simulink model "Roll_Autopilot_PP"  (R2017b)
settings: Solver=FixedStepDiscrete  StartTime=0.0  StopTime=10.0  FixedStep=0.025000  RelTol=1e-3
model workspace (MAT data in the model file):
  MCOS : class17 (value not decoded)
  already_pp = 1
  compositionalMap : struct (value not decoded)
  MCOS : class17 (value not decoded)
  MCOS : class17 (value not decoded)
  verificationResults : struct (value not decoded)
undefined symbols (not defined in the file): contractAfterSimulation, contractBeforeSimulation, ContractBlock, ContractEnsureBlock, ContractGuaranteeBlock, ContractModeBlock, ContractRequireBlock, ContractValidatorBlock, pp_lib, saturation, saveValidatorParameters, slcm, Ts
(part 3 of 3)

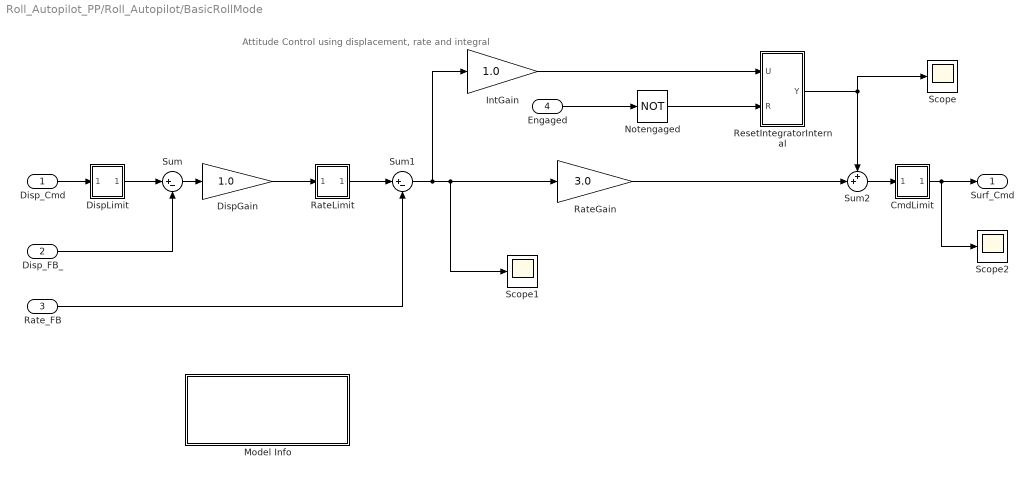
== system Roll_Autopilot_PP/Roll_Autopilot/BasicRollMode ==
  note: Attitude Control using displacement, rate and integral
  Disp_Cmd : Inport  OutDataTypeStr=double  PortDimensions=1
  Disp_FB_ : Inport  Port=2  OutDataTypeStr=double  PortDimensions=1  SampleTime=1/40
  Rate_FB : Inport  Port=3  OutDataTypeStr=double  PortDimensions=1  SampleTime=1/40
  Engaged : Inport  Port=4  OutDataTypeStr=boolean  PortDimensions=1  SampleTime=1/40
  CmdLimit : Subsystem  AncestorBlock=pp_lib/saturation  TreatAsAtomicUnit=on
  DispGain : Gain  Gain=1.0
  DispLimit : Subsystem  AncestorBlock=pp_lib/saturation  TreatAsAtomicUnit=on
  IntGain : Gain  Gain=1.0
  Model Info : Subsystem  AncestorBlock=simulink/Model-Wide Utilities/Model Info  LoadFcn=slcm LoadBlock;  InitFcn=slcm('UpdateAllCMBlocksInThisModelInit')  TreatAsAtomicUnit=on  mask(CMBlock){Frame=on, DisplayStringWithTags=|, MaskDisplayString=Attitude Controller\nAuthor: hbourbou\nVersion: 1.13\nDate: Wed Nov 06 15:53:17 2019, HorizontalTextAlignment=Left, LeftAlignmentValue=0.02}
      mask DisplayStringWithTags=|
      | Attitude Controller
      | Author: %<LastModifiedBy>
      | Version: %<ModelVersion>
      | Date: %<LastModificationDate>
      mask prompts: Frame "Simulink:masks:Frame_MP"; DisplayStringWithTags "Simulink:masks:DisplayStringWithTags_MP"; MaskDisplayString "Simulink:masks:MaskDisplayString_MP"; HorizontalTextAlignment "Simulink:masks:HorizontalTextAlignment_MP"; LeftAlignmentValue "Simulink:masks:LeftAlignmentValue_MP"
      mask help: Simulink:masks:CMBlock_MD
      settings: CopyFcn=slcm CopyBlock;  DeleteFcn=slcm Cancel;  PostSaveFcn=slcm('UpdateAllCMBlocksInThisModel')  NameChangeFcn=slcm Rename;  OpenFcn=slcm
      mask Display: text(slResolve(LeftAlignmentValue, gcbh), 0.5, MaskDisplayString, 'HorizontalAlignment', HorizontalTextAlignment)
  Notengaged : Logic  Operator=NOT  IconShape=distinctive  AllPortsSameDT=off  OutDataTypeStr=boolean
  RateGain : Gain  Gain=3.0
  RateLimit : Subsystem  AncestorBlock=pp_lib/saturation  TreatAsAtomicUnit=on
  ResetIntegratorInternal : Subsystem  TreatAsAtomicUnit=on
  Scope : Scope
  Scope1 : Scope
  Scope2 : Scope
  Sum : Sum  Inputs=|+-
  Sum1 : Sum  Inputs=|+-
  Sum2 : Sum  Inputs=++|
  Surf_Cmd : Outport  OutDataTypeStr=double  PortDimensions=1  SampleTime=1/40  VectorParamsAs1DForOutWhenUnconnected=off
  wires:
  Engaged/1 -> Notengaged/1
  Disp_Cmd/1 -> DispLimit/1(In)
  RateLimit/1(Out) -> Sum1/1
  ResetIntegratorInternal/1(Y) -> Sum2/1, Scope/1
  Notengaged/1 -> ResetIntegratorInternal/2(R)
  Rate_FB/1 -> Sum1/2
  Sum1/1 -> IntGain/1, Scope1/1, RateGain/1
  CmdLimit/1(Out) -> Scope2/1, Surf_Cmd/1
  RateGain/1 -> Sum2/2
  DispGain/1 -> RateLimit/1(In)
  Sum/1 -> DispGain/1
  Disp_FB_/1 -> Sum/2
  DispLimit/1(Out) -> Sum/1
  Sum2/1 -> CmdLimit/1(In)
  IntGain/1 -> ResetIntegratorInternal/1(U)

== system Roll_Autopilot_PP/Roll_Autopilot/HeadingMode ==
  PsiRef : Inport  OutDataTypeStr=double  PortDimensions=1  SampleTime=1/40  Interpolate=off
  Psi : Inport  Port=2  OutDataTypeStr=double  PortDimensions=1  SampleTime=1/40  Interpolate=off
  TAS : Inport  Port=3  OutDataTypeStr=double  PortDimensions=1  SampleTime=1/40  Interpolate=off
  DispGain : Gain  Gain=0.015
  Model Info : Subsystem  AncestorBlock=simulink/Model-Wide Utilities/Model Info  LoadFcn=slcm LoadBlock;  InitFcn=slcm('UpdateAllCMBlocksInThisModelInit')  TreatAsAtomicUnit=on  mask(CMBlock){Frame=on, DisplayStringWithTags=|, MaskDisplayString=Heading Mode\nAuthor: hbourbou\nVersion: 1.13\nDate: Wed Nov 06 15:53:17 2019, HorizontalTextAlignment=Left, LeftAlignmentValue=0.02}
      mask DisplayStringWithTags=|
      | Heading Mode
      | Author: %<LastModifiedBy>
      | Version: %<ModelVersion>
      | Date: %<LastModificationDate>
      mask prompts: Frame "Simulink:masks:Frame_MP"; DisplayStringWithTags "Simulink:masks:DisplayStringWithTags_MP"; MaskDisplayString "Simulink:masks:MaskDisplayString_MP"; HorizontalTextAlignment "Simulink:masks:HorizontalTextAlignment_MP"; LeftAlignmentValue "Simulink:masks:LeftAlignmentValue_MP"
      mask help: Simulink:masks:CMBlock_MD
      settings: CopyFcn=slcm CopyBlock;  DeleteFcn=slcm Cancel;  PostSaveFcn=slcm('UpdateAllCMBlocksInThisModel')  NameChangeFcn=slcm Rename;  OpenFcn=slcm
      mask Display: text(slResolve(LeftAlignmentValue, gcbh), 0.5, MaskDisplayString, 'HorizontalAlignment', HorizontalTextAlignment)
  Product : Product  RndMeth=Zero
  anglediff : Subsystem  TreatAsAtomicUnit=on
  PhiCmd : Outport  OutDataTypeStr=double  PortDimensions=1  SampleTime=1/40  VectorParamsAs1DForOutWhenUnconnected=off
  wires:
  PsiRef/1 -> anglediff/1(plus)
  anglediff/1(diff) -> DispGain/1  "hdgError"
  TAS/1 -> Product/2
  DispGain/1 -> Product/1
  Psi/1 -> anglediff/2(minus)
  Product/1 -> PhiCmd/1

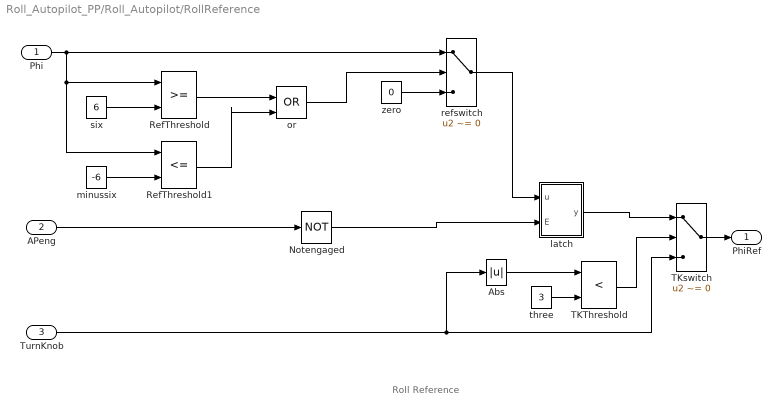
== system Roll_Autopilot_PP/Roll_Autopilot/RollReference ==
  note: Roll Reference
  Phi : Inport
  APeng : Inport  Port=2
  TurnKnob : Inport  Port=3
  Abs : Abs
  Notengaged : Logic  Operator=NOT  IconShape=distinctive  AllPortsSameDT=off  OutDataTypeStr=boolean
  RefThreshold : RelationalOperator  OutDataTypeStr=boolean  RndMeth=Nearest  InputSameDT=on
  RefThreshold1 : RelationalOperator  Operator=<=  OutDataTypeStr=boolean  RndMeth=Nearest  InputSameDT=on
  TKThreshold : RelationalOperator  Operator=<  OutDataTypeStr=boolean  RndMeth=Nearest  InputSameDT=on
  TKswitch : Switch  Criteria=u2 ~= 0
  latch : Subsystem  TreatAsAtomicUnit=on
  minussix : Constant  Value=-6
  or : Logic  Operator=OR  IconShape=distinctive  OutDataTypeStr=boolean
  refswitch : Switch  Criteria=u2 ~= 0
  six : Constant  Value=6
  three : Constant  Value=3  OutDataTypeStr=double
  zero : Constant  Value=0
  PhiRef : Outport  VectorParamsAs1DForOutWhenUnconnected=off
  wires:
  minussix/1 -> RefThreshold1/2
  RefThreshold1/1 -> or/2
  RefThreshold/1 -> or/1
  or/1 -> refswitch/2
  zero/1 -> refswitch/3
  six/1 -> RefThreshold/2
  TKswitch/1 -> PhiRef/1
  APeng/1 -> Notengaged/1
  Phi/1 -> RefThreshold1/1, RefThreshold/1, refswitch/1
  Abs/1 -> TKThreshold/1
  three/1 -> TKThreshold/2
  TurnKnob/1 -> Abs/1, TKswitch/3
  TKThreshold/1 -> TKswitch/2
  latch/1(y) -> TKswitch/1
  refswitch/1 -> latch/1(u)
  Notengaged/1 -> latch/2(E)

== system Roll_Autopilot_PP/Roll_Autopilot_RollAutopilotSpec1/AP_minus_001 ==
  In1 : Inport
  guarantee : Outport  OutDataTypeStr=boolean
  wires:
  In1/1 -> guarantee/1

== system Roll_Autopilot_PP/Roll_Autopilot_RollAutopilotSpec1/AP_minus_003A ==
  In1 : Inport
  guarantee : Outport  OutDataTypeStr=boolean
  wires:
  In1/1 -> guarantee/1

== system Roll_Autopilot_PP/Roll_Autopilot_RollAutopilotSpec1/AP_minus_003B ==
  In1 : Inport
  guarantee : Outport  OutDataTypeStr=boolean
  wires:
  In1/1 -> guarantee/1

== system Roll_Autopilot_PP/Roll_Autopilot_RollAutopilotSpec1/AP_minus_003C ==
  In1 : Inport
  guarantee : Outport  OutDataTypeStr=boolean
  wires:
  In1/1 -> guarantee/1

== system Roll_Autopilot_PP/Roll_Autopilot_RollAutopilotSpec1/AP_minus_003D ==
  In1 : Inport
  guarantee : Outport  OutDataTypeStr=boolean
  wires:
  In1/1 -> guarantee/1

== system Roll_Autopilot_PP/Roll_Autopilot_RollAutopilotSpec1/AP_minus_007 ==
  In1 : Inport
  guarantee : Outport  OutDataTypeStr=boolean
  wires:
  In1/1 -> guarantee/1

== system Roll_Autopilot_PP/Roll_Autopilot_RollAutopilotSpec1/H_call ==
  H_X : Inport  OutDataTypeStr=boolean
  Arrow_xxH_1_ni_23 : Delay  DelayLength=1  InitialCondition=1
  PRE_xxH_2 : Delay  DelayLength=1  InitialCondition=0
  branch_6_IF : Switch  Criteria=u2 ~= 0
  xxH_1_ni_23_init : Constant  Value=0  OutDataTypeStr=boolean
  xxH_3_operator : Logic  AllPortsSameDT=off  OutDataTypeStr=boolean
  H_Y : Outport
  wires:
  PRE_xxH_2/1 -> xxH_3_operator/2
  xxH_3_operator/1 -> branch_6_IF/3
  Arrow_xxH_1_ni_23/1 -> branch_6_IF/2
  xxH_1_ni_23_init/1 -> Arrow_xxH_1_ni_23/1
  branch_6_IF/1 -> H_Y/1, PRE_xxH_2/1
  H_X/1 -> xxH_3_operator/1, branch_6_IF/1

== system Roll_Autopilot_PP/Roll_Autopilot_RollAutopilotSpec1/H_call1 ==
  H_X : Inport  OutDataTypeStr=boolean
  Arrow_xxH_1_ni_23 : Delay  DelayLength=1  InitialCondition=1
  PRE_xxH_2 : Delay  DelayLength=1  InitialCondition=0
  branch_6_IF : Switch  Criteria=u2 ~= 0
  xxH_1_ni_23_init : Constant  Value=0  OutDataTypeStr=boolean
  xxH_3_operator : Logic  AllPortsSameDT=off  OutDataTypeStr=boolean
  H_Y : Outport
  wires:
  PRE_xxH_2/1 -> xxH_3_operator/2
  xxH_3_operator/1 -> branch_6_IF/3
  Arrow_xxH_1_ni_23/1 -> branch_6_IF/2
  xxH_1_ni_23_init/1 -> Arrow_xxH_1_ni_23/1
  branch_6_IF/1 -> H_Y/1, PRE_xxH_2/1
  H_X/1 -> xxH_3_operator/1, branch_6_IF/1

== system Roll_Autopilot_PP/Roll_Autopilot_RollAutopilotSpec1/H_call11 ==
  H_X : Inport  OutDataTypeStr=boolean
  Arrow_xxH_1_ni_23 : Delay  DelayLength=1  InitialCondition=1
  PRE_xxH_2 : Delay  DelayLength=1  InitialCondition=0
  branch_6_IF : Switch  Criteria=u2 ~= 0
  xxH_1_ni_23_init : Constant  Value=0  OutDataTypeStr=boolean
  xxH_3_operator : Logic  AllPortsSameDT=off  OutDataTypeStr=boolean
  H_Y : Outport
  wires:
  PRE_xxH_2/1 -> xxH_3_operator/2
  xxH_3_operator/1 -> branch_6_IF/3
  Arrow_xxH_1_ni_23/1 -> branch_6_IF/2
  xxH_1_ni_23_init/1 -> Arrow_xxH_1_ni_23/1
  branch_6_IF/1 -> H_Y/1, PRE_xxH_2/1
  H_X/1 -> xxH_3_operator/1, branch_6_IF/1

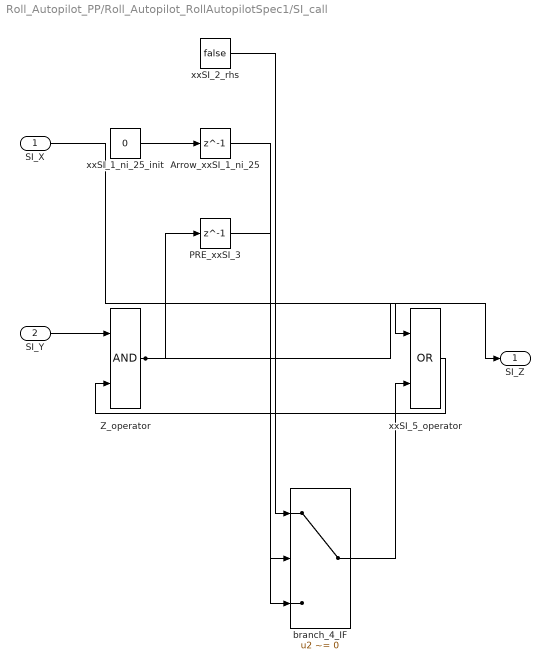
== system Roll_Autopilot_PP/Roll_Autopilot_RollAutopilotSpec1/SI_call ==
  SI_X : Inport  OutDataTypeStr=boolean
  SI_Y : Inport  Port=2  OutDataTypeStr=boolean
  Arrow_xxSI_1_ni_25 : Delay  DelayLength=1  InitialCondition=1
  PRE_xxSI_3 : Delay  DelayLength=1  InitialCondition=0
  Z_operator : Logic  AllPortsSameDT=off  OutDataTypeStr=boolean
  branch_4_IF : Switch  Criteria=u2 ~= 0
  xxSI_1_ni_25_init : Constant  Value=0  OutDataTypeStr=boolean
  xxSI_2_rhs : Constant  Value=false  OutDataTypeStr=boolean
  xxSI_5_operator : Logic  Operator=OR  AllPortsSameDT=off  OutDataTypeStr=boolean
  SI_Z : Outport
  wires:
  branch_4_IF/1 -> xxSI_5_operator/2
  SI_X/1 -> xxSI_5_operator/1
  PRE_xxSI_3/1 -> branch_4_IF/3
  Arrow_xxSI_1_ni_25/1 -> branch_4_IF/2
  xxSI_2_rhs/1 -> branch_4_IF/1
  xxSI_5_operator/1 -> Z_operator/2
  SI_Y/1 -> Z_operator/1
  xxSI_1_ni_25_init/1 -> Arrow_xxSI_1_ni_25/1
  Z_operator/1 -> SI_Z/1, PRE_xxSI_3/1

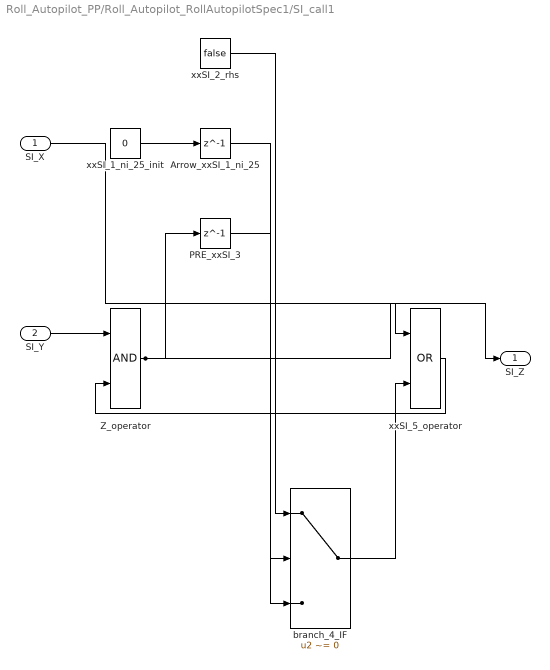
== system Roll_Autopilot_PP/Roll_Autopilot_RollAutopilotSpec1/SI_call1 ==
  SI_X : Inport  OutDataTypeStr=boolean
  SI_Y : Inport  Port=2  OutDataTypeStr=boolean
  Arrow_xxSI_1_ni_25 : Delay  DelayLength=1  InitialCondition=1
  PRE_xxSI_3 : Delay  DelayLength=1  InitialCondition=0
  Z_operator : Logic  AllPortsSameDT=off  OutDataTypeStr=boolean
  branch_4_IF : Switch  Criteria=u2 ~= 0
  xxSI_1_ni_25_init : Constant  Value=0  OutDataTypeStr=boolean
  xxSI_2_rhs : Constant  Value=false  OutDataTypeStr=boolean
  xxSI_5_operator : Logic  Operator=OR  AllPortsSameDT=off  OutDataTypeStr=boolean
  SI_Z : Outport
  wires:
  branch_4_IF/1 -> xxSI_5_operator/2
  SI_X/1 -> xxSI_5_operator/1
  PRE_xxSI_3/1 -> branch_4_IF/3
  Arrow_xxSI_1_ni_25/1 -> branch_4_IF/2
  xxSI_2_rhs/1 -> branch_4_IF/1
  xxSI_5_operator/1 -> Z_operator/2
  SI_Y/1 -> Z_operator/1
  xxSI_1_ni_25_init/1 -> Arrow_xxSI_1_ni_25/1
  Z_operator/1 -> SI_Z/1, PRE_xxSI_3/1

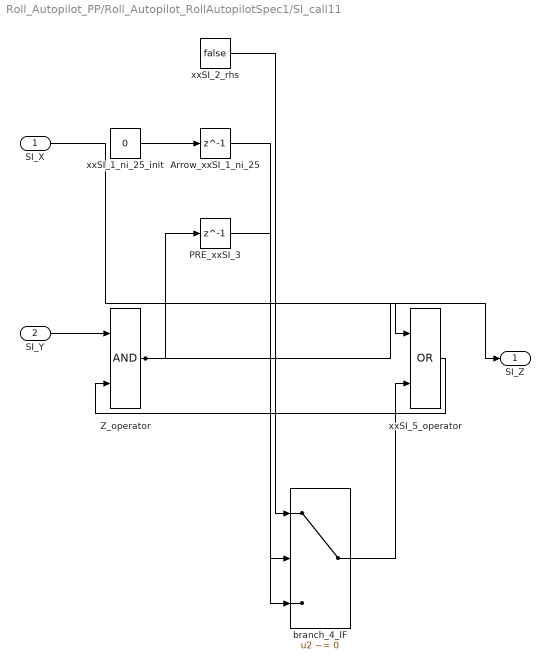
== system Roll_Autopilot_PP/Roll_Autopilot_RollAutopilotSpec1/SI_call11 ==
  SI_X : Inport  OutDataTypeStr=boolean
  SI_Y : Inport  Port=2  OutDataTypeStr=boolean
  Arrow_xxSI_1_ni_25 : Delay  DelayLength=1  InitialCondition=1
  PRE_xxSI_3 : Delay  DelayLength=1  InitialCondition=0
  Z_operator : Logic  AllPortsSameDT=off  OutDataTypeStr=boolean
  branch_4_IF : Switch  Criteria=u2 ~= 0
  xxSI_1_ni_25_init : Constant  Value=0  OutDataTypeStr=boolean
  xxSI_2_rhs : Constant  Value=false  OutDataTypeStr=boolean
  xxSI_5_operator : Logic  Operator=OR  AllPortsSameDT=off  OutDataTypeStr=boolean
  SI_Z : Outport
  wires:
  branch_4_IF/1 -> xxSI_5_operator/2
  SI_X/1 -> xxSI_5_operator/1
  PRE_xxSI_3/1 -> branch_4_IF/3
  Arrow_xxSI_1_ni_25/1 -> branch_4_IF/2
  xxSI_2_rhs/1 -> branch_4_IF/1
  xxSI_5_operator/1 -> Z_operator/2
  SI_Y/1 -> Z_operator/1
  xxSI_1_ni_25_init/1 -> Arrow_xxSI_1_ni_25/1
  Z_operator/1 -> SI_Z/1, PRE_xxSI_3/1

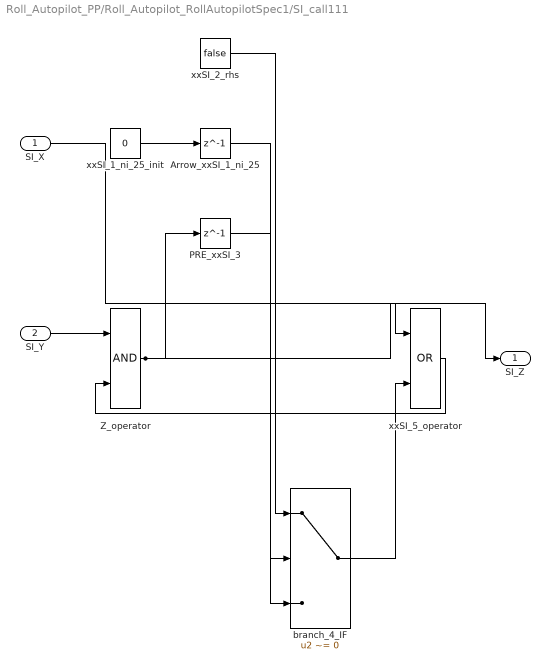
== system Roll_Autopilot_PP/Roll_Autopilot_RollAutopilotSpec1/SI_call111 ==
  SI_X : Inport  OutDataTypeStr=boolean
  SI_Y : Inport  Port=2  OutDataTypeStr=boolean
  Arrow_xxSI_1_ni_25 : Delay  DelayLength=1  InitialCondition=1
  PRE_xxSI_3 : Delay  DelayLength=1  InitialCondition=0
  Z_operator : Logic  AllPortsSameDT=off  OutDataTypeStr=boolean
  branch_4_IF : Switch  Criteria=u2 ~= 0
  xxSI_1_ni_25_init : Constant  Value=0  OutDataTypeStr=boolean
  xxSI_2_rhs : Constant  Value=false  OutDataTypeStr=boolean
  xxSI_5_operator : Logic  Operator=OR  AllPortsSameDT=off  OutDataTypeStr=boolean
  SI_Z : Outport
  wires:
  branch_4_IF/1 -> xxSI_5_operator/2
  SI_X/1 -> xxSI_5_operator/1
  PRE_xxSI_3/1 -> branch_4_IF/3
  Arrow_xxSI_1_ni_25/1 -> branch_4_IF/2
  xxSI_2_rhs/1 -> branch_4_IF/1
  xxSI_5_operator/1 -> Z_operator/2
  SI_Y/1 -> Z_operator/1
  xxSI_1_ni_25_init/1 -> Arrow_xxSI_1_ni_25/1
  Z_operator/1 -> SI_Z/1, PRE_xxSI_3/1

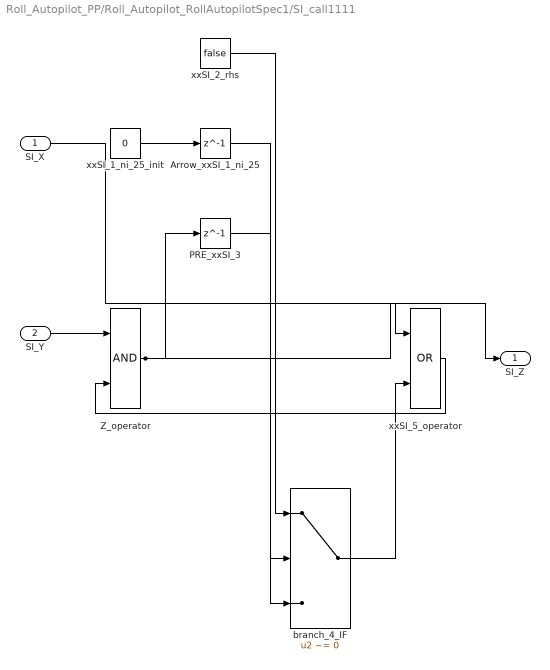
== system Roll_Autopilot_PP/Roll_Autopilot_RollAutopilotSpec1/SI_call1111 ==
  SI_X : Inport  OutDataTypeStr=boolean
  SI_Y : Inport  Port=2  OutDataTypeStr=boolean
  Arrow_xxSI_1_ni_25 : Delay  DelayLength=1  InitialCondition=1
  PRE_xxSI_3 : Delay  DelayLength=1  InitialCondition=0
  Z_operator : Logic  AllPortsSameDT=off  OutDataTypeStr=boolean
  branch_4_IF : Switch  Criteria=u2 ~= 0
  xxSI_1_ni_25_init : Constant  Value=0  OutDataTypeStr=boolean
  xxSI_2_rhs : Constant  Value=false  OutDataTypeStr=boolean
  xxSI_5_operator : Logic  Operator=OR  AllPortsSameDT=off  OutDataTypeStr=boolean
  SI_Z : Outport
  wires:
  branch_4_IF/1 -> xxSI_5_operator/2
  SI_X/1 -> xxSI_5_operator/1
  PRE_xxSI_3/1 -> branch_4_IF/3
  Arrow_xxSI_1_ni_25/1 -> branch_4_IF/2
  xxSI_2_rhs/1 -> branch_4_IF/1
  xxSI_5_operator/1 -> Z_operator/2
  SI_Y/1 -> Z_operator/1
  xxSI_1_ni_25_init/1 -> Arrow_xxSI_1_ni_25/1
  Z_operator/1 -> SI_Z/1, PRE_xxSI_3/1

== system Roll_Autopilot_PP/Roll_Autopilot_RollAutopilotSpec1/SI_call11111 ==
  SI_X : Inport  OutDataTypeStr=boolean
  SI_Y : Inport  Port=2  OutDataTypeStr=boolean
  Arrow_xxSI_1_ni_25 : Delay  DelayLength=1  InitialCondition=1
  PRE_xxSI_3 : Delay  DelayLength=1  InitialCondition=0
  Z_operator : Logic  AllPortsSameDT=off  OutDataTypeStr=boolean
  branch_4_IF : Switch  Criteria=u2 ~= 0
  xxSI_1_ni_25_init : Constant  Value=0  OutDataTypeStr=boolean
  xxSI_2_rhs : Constant  Value=false  OutDataTypeStr=boolean
  xxSI_5_operator : Logic  Operator=OR  AllPortsSameDT=off  OutDataTypeStr=boolean
  SI_Z : Outport
  wires:
  branch_4_IF/1 -> xxSI_5_operator/2
  SI_X/1 -> xxSI_5_operator/1
  PRE_xxSI_3/1 -> branch_4_IF/3
  Arrow_xxSI_1_ni_25/1 -> branch_4_IF/2
  xxSI_2_rhs/1 -> branch_4_IF/1
  xxSI_5_operator/1 -> Z_operator/2
  SI_Y/1 -> Z_operator/1
  xxSI_1_ni_25_init/1 -> Arrow_xxSI_1_ni_25/1
  Z_operator/1 -> SI_Z/1, PRE_xxSI_3/1

== system Roll_Autopilot_PP/Roll_Autopilot_RollAutopilotSpec1/SI_call111111 ==
  SI_X : Inport  OutDataTypeStr=boolean
  SI_Y : Inport  Port=2  OutDataTypeStr=boolean
  Arrow_xxSI_1_ni_25 : Delay  DelayLength=1  InitialCondition=1
  PRE_xxSI_3 : Delay  DelayLength=1  InitialCondition=0
  Z_operator : Logic  AllPortsSameDT=off  OutDataTypeStr=boolean
  branch_4_IF : Switch  Criteria=u2 ~= 0
  xxSI_1_ni_25_init : Constant  Value=0  OutDataTypeStr=boolean
  xxSI_2_rhs : Constant  Value=false  OutDataTypeStr=boolean
  xxSI_5_operator : Logic  Operator=OR  AllPortsSameDT=off  OutDataTypeStr=boolean
  SI_Z : Outport
  wires:
  branch_4_IF/1 -> xxSI_5_operator/2
  SI_X/1 -> xxSI_5_operator/1
  PRE_xxSI_3/1 -> branch_4_IF/3
  Arrow_xxSI_1_ni_25/1 -> branch_4_IF/2
  xxSI_2_rhs/1 -> branch_4_IF/1
  xxSI_5_operator/1 -> Z_operator/2
  SI_Y/1 -> Z_operator/1
  xxSI_1_ni_25_init/1 -> Arrow_xxSI_1_ni_25/1
  Z_operator/1 -> SI_Z/1, PRE_xxSI_3/1

== system Roll_Autopilot_PP/Roll_Autopilot_RollAutopilotSpec1/SI_call1111111 ==
  SI_X : Inport  OutDataTypeStr=boolean
  SI_Y : Inport  Port=2  OutDataTypeStr=boolean
  Arrow_xxSI_1_ni_25 : Delay  DelayLength=1  InitialCondition=1
  PRE_xxSI_3 : Delay  DelayLength=1  InitialCondition=0
  Z_operator : Logic  AllPortsSameDT=off  OutDataTypeStr=boolean
  branch_4_IF : Switch  Criteria=u2 ~= 0
  xxSI_1_ni_25_init : Constant  Value=0  OutDataTypeStr=boolean
  xxSI_2_rhs : Constant  Value=false  OutDataTypeStr=boolean
  xxSI_5_operator : Logic  Operator=OR  AllPortsSameDT=off  OutDataTypeStr=boolean
  SI_Z : Outport
  wires:
  branch_4_IF/1 -> xxSI_5_operator/2
  SI_X/1 -> xxSI_5_operator/1
  PRE_xxSI_3/1 -> branch_4_IF/3
  Arrow_xxSI_1_ni_25/1 -> branch_4_IF/2
  xxSI_2_rhs/1 -> branch_4_IF/1
  xxSI_5_operator/1 -> Z_operator/2
  SI_Y/1 -> Z_operator/1
  xxSI_1_ni_25_init/1 -> Arrow_xxSI_1_ni_25/1
  Z_operator/1 -> SI_Z/1, PRE_xxSI_3/1

== system Roll_Autopilot_PP/Roll_Autopilot_RollAutopilotSpec1/SI_call11111111 ==
  SI_X : Inport  OutDataTypeStr=boolean
  SI_Y : Inport  Port=2  OutDataTypeStr=boolean
  Arrow_xxSI_1_ni_25 : Delay  DelayLength=1  InitialCondition=1
  PRE_xxSI_3 : Delay  DelayLength=1  InitialCondition=0
  Z_operator : Logic  AllPortsSameDT=off  OutDataTypeStr=boolean
  branch_4_IF : Switch  Criteria=u2 ~= 0
  xxSI_1_ni_25_init : Constant  Value=0  OutDataTypeStr=boolean
  xxSI_2_rhs : Constant  Value=false  OutDataTypeStr=boolean
  xxSI_5_operator : Logic  Operator=OR  AllPortsSameDT=off  OutDataTypeStr=boolean
  SI_Z : Outport
  wires:
  branch_4_IF/1 -> xxSI_5_operator/2
  SI_X/1 -> xxSI_5_operator/1
  PRE_xxSI_3/1 -> branch_4_IF/3
  Arrow_xxSI_1_ni_25/1 -> branch_4_IF/2
  xxSI_2_rhs/1 -> branch_4_IF/1
  xxSI_5_operator/1 -> Z_operator/2
  SI_Y/1 -> Z_operator/1
  xxSI_1_ni_25_init/1 -> Arrow_xxSI_1_ni_25/1
  Z_operator/1 -> SI_Z/1, PRE_xxSI_3/1

== system Roll_Autopilot_PP/Roll_Autopilot_RollAutopilotSpec1/hdg_hold_mode ==
  note: Shouldn't not be edited
  require : Inport  OutDataTypeStr=boolean
  ensure : Inport  Port=2  OutDataTypeStr=boolean
  and : Logic  Operator=NOT  IconShape=distinctive  AllPortsSameDT=off  OutDataTypeStr=boolean
  or : Logic  Operator=OR  IconShape=distinctive  AllPortsSameDT=off  OutDataTypeStr=boolean
  mode : Outport
  wires:
  or/1 -> mode/1
  ensure/1 -> or/2
  and/1 -> or/1
  require/1 -> and/1

== system Roll_Autopilot_PP/Roll_Autopilot_RollAutopilotSpec1/hdg_hold_mode_ensure ==
  In1 : Inport
  ensure : Outport  OutDataTypeStr=boolean
  wires:
  In1/1 -> ensure/1

== system Roll_Autopilot_PP/Roll_Autopilot_RollAutopilotSpec1/hdg_hold_mode_require ==
  In1 : Inport
  require : Outport  OutDataTypeStr=boolean
  wires:
  In1/1 -> require/1

== system Roll_Autopilot_PP/Roll_Autopilot_RollAutopilotSpec1/roll_hold_mode ==
  note: Shouldn't not be edited
  require : Inport  OutDataTypeStr=boolean
  ensure : Inport  Port=2  OutDataTypeStr=boolean
  and : Logic  Operator=NOT  IconShape=distinctive  AllPortsSameDT=off  OutDataTypeStr=boolean
  or : Logic  Operator=OR  IconShape=distinctive  AllPortsSameDT=off  OutDataTypeStr=boolean
  mode : Outport
  wires:
  or/1 -> mode/1
  ensure/1 -> or/2
  and/1 -> or/1
  require/1 -> and/1

== system Roll_Autopilot_PP/Roll_Autopilot_RollAutopilotSpec1/roll_hold_mode_ensure ==
  In1 : Inport
  ensure : Outport  OutDataTypeStr=boolean
  wires:
  In1/1 -> ensure/1

== system Roll_Autopilot_PP/Roll_Autopilot_RollAutopilotSpec1/roll_hold_mode_require ==
  In1 : Inport
  require : Outport  OutDataTypeStr=boolean
  wires:
  In1/1 -> require/1

== system Roll_Autopilot_PP/Roll_Autopilot_RollAutopilotSpec1/spec206_operator ==
  A : Inport
  B : Inport  Port=2
  Logical_newline_Operator : Logic  Operator=OR  AllPortsSameDT=off  OutDataTypeStr=boolean
  Logical_newline_Operator1 : Logic  Operator=NOT  AllPortsSameDT=off  OutDataTypeStr=boolean
  A_equal__equal__gt_B : Outport  VectorParamsAs1DForOutWhenUnconnected=off
  wires:
  Logical_newline_Operator1/1 -> Logical_newline_Operator/1
  Logical_newline_Operator/1 -> A_equal__equal__gt_B/1
  A/1 -> Logical_newline_Operator1/1
  B/1 -> Logical_newline_Operator/2

== system Roll_Autopilot_PP/Roll_Autopilot_RollAutopilotSpec1/spec252_operator ==
  A : Inport
  B : Inport  Port=2
  Logical_newline_Operator : Logic  Operator=OR  AllPortsSameDT=off  OutDataTypeStr=boolean
  Logical_newline_Operator1 : Logic  Operator=NOT  AllPortsSameDT=off  OutDataTypeStr=boolean
  A_equal__equal__gt_B : Outport  VectorParamsAs1DForOutWhenUnconnected=off
  wires:
  Logical_newline_Operator1/1 -> Logical_newline_Operator/1
  Logical_newline_Operator/1 -> A_equal__equal__gt_B/1
  A/1 -> Logical_newline_Operator1/1
  B/1 -> Logical_newline_Operator/2

== system Roll_Autopilot_PP/Roll_Autopilot_RollAutopilotSpec1/xxRollAutopilotSpec_107_operator ==
  A : Inport
  B : Inport  Port=2
  Logical_newline_Operator : Logic  Operator=OR  AllPortsSameDT=off  OutDataTypeStr=boolean
  Logical_newline_Operator1 : Logic  Operator=NOT  AllPortsSameDT=off  OutDataTypeStr=boolean
  A_equal__equal__gt_B : Outport  VectorParamsAs1DForOutWhenUnconnected=off
  wires:
  Logical_newline_Operator1/1 -> Logical_newline_Operator/1
  Logical_newline_Operator/1 -> A_equal__equal__gt_B/1
  A/1 -> Logical_newline_Operator1/1
  B/1 -> Logical_newline_Operator/2

== system Roll_Autopilot_PP/Roll_Autopilot_RollAutopilotSpec1/xxRollAutopilotSpec_112_operator ==
  A : Inport
  B : Inport  Port=2
  Logical_newline_Operator : Logic  Operator=OR  AllPortsSameDT=off  OutDataTypeStr=boolean
  Logical_newline_Operator1 : Logic  Operator=NOT  AllPortsSameDT=off  OutDataTypeStr=boolean
  A_equal__equal__gt_B : Outport  VectorParamsAs1DForOutWhenUnconnected=off
  wires:
  Logical_newline_Operator1/1 -> Logical_newline_Operator/1
  Logical_newline_Operator/1 -> A_equal__equal__gt_B/1
  A/1 -> Logical_newline_Operator1/1
  B/1 -> Logical_newline_Operator/2

== system Roll_Autopilot_PP/Roll_Autopilot_RollAutopilotSpec1/xxRollAutopilotSpec_11_operator ==
  A : Inport
  B : Inport  Port=2
  Logical_newline_Operator : Logic  Operator=OR  AllPortsSameDT=off  OutDataTypeStr=boolean
  Logical_newline_Operator1 : Logic  Operator=NOT  AllPortsSameDT=off  OutDataTypeStr=boolean
  A_equal__equal__gt_B : Outport  VectorParamsAs1DForOutWhenUnconnected=off
  wires:
  Logical_newline_Operator1/1 -> Logical_newline_Operator/1
  Logical_newline_Operator/1 -> A_equal__equal__gt_B/1
  A/1 -> Logical_newline_Operator1/1
  B/1 -> Logical_newline_Operator/2

== system Roll_Autopilot_PP/Roll_Autopilot_RollAutopilotSpec1/xxRollAutopilotSpec_127_operator ==
  A : Inport
  B : Inport  Port=2
  Logical_newline_Operator : Logic  Operator=OR  AllPortsSameDT=off  OutDataTypeStr=boolean
  Logical_newline_Operator1 : Logic  Operator=NOT  AllPortsSameDT=off  OutDataTypeStr=boolean
  A_equal__equal__gt_B : Outport  VectorParamsAs1DForOutWhenUnconnected=off
  wires:
  Logical_newline_Operator1/1 -> Logical_newline_Operator/1
  Logical_newline_Operator/1 -> A_equal__equal__gt_B/1
  A/1 -> Logical_newline_Operator1/1
  B/1 -> Logical_newline_Operator/2

== system Roll_Autopilot_PP/Roll_Autopilot_RollAutopilotSpec1/xxRollAutopilotSpec_131_operator ==
  A : Inport
  B : Inport  Port=2
  Logical_newline_Operator : Logic  Operator=OR  AllPortsSameDT=off  OutDataTypeStr=boolean
  Logical_newline_Operator1 : Logic  Operator=NOT  AllPortsSameDT=off  OutDataTypeStr=boolean
  A_equal__equal__gt_B : Outport  VectorParamsAs1DForOutWhenUnconnected=off
  wires:
  Logical_newline_Operator1/1 -> Logical_newline_Operator/1
  Logical_newline_Operator/1 -> A_equal__equal__gt_B/1
  A/1 -> Logical_newline_Operator1/1
  B/1 -> Logical_newline_Operator/2

== system Roll_Autopilot_PP/Roll_Autopilot_RollAutopilotSpec1/xxRollAutopilotSpec_136_operator ==
  A : Inport
  B : Inport  Port=2
  Logical_newline_Operator : Logic  Operator=OR  AllPortsSameDT=off  OutDataTypeStr=boolean
  Logical_newline_Operator1 : Logic  Operator=NOT  AllPortsSameDT=off  OutDataTypeStr=boolean
  A_equal__equal__gt_B : Outport  VectorParamsAs1DForOutWhenUnconnected=off
  wires:
  Logical_newline_Operator1/1 -> Logical_newline_Operator/1
  Logical_newline_Operator/1 -> A_equal__equal__gt_B/1
  A/1 -> Logical_newline_Operator1/1
  B/1 -> Logical_newline_Operator/2

== system Roll_Autopilot_PP/Roll_Autopilot_RollAutopilotSpec1/xxRollAutopilotSpec_148_operator ==
  A : Inport
  B : Inport  Port=2
  Logical_newline_Operator : Logic  Operator=OR  AllPortsSameDT=off  OutDataTypeStr=boolean
  Logical_newline_Operator1 : Logic  Operator=NOT  AllPortsSameDT=off  OutDataTypeStr=boolean
  A_equal__equal__gt_B : Outport  VectorParamsAs1DForOutWhenUnconnected=off
  wires:
  Logical_newline_Operator1/1 -> Logical_newline_Operator/1
  Logical_newline_Operator/1 -> A_equal__equal__gt_B/1
  A/1 -> Logical_newline_Operator1/1
  B/1 -> Logical_newline_Operator/2

== system Roll_Autopilot_PP/Roll_Autopilot_RollAutopilotSpec1/xxRollAutopilotSpec_26_operator ==
  A : Inport
  B : Inport  Port=2
  Logical_newline_Operator : Logic  Operator=OR  AllPortsSameDT=off  OutDataTypeStr=boolean
  Logical_newline_Operator1 : Logic  Operator=NOT  AllPortsSameDT=off  OutDataTypeStr=boolean
  A_equal__equal__gt_B : Outport  VectorParamsAs1DForOutWhenUnconnected=off
  wires:
  Logical_newline_Operator1/1 -> Logical_newline_Operator/1
  Logical_newline_Operator/1 -> A_equal__equal__gt_B/1
  A/1 -> Logical_newline_Operator1/1
  B/1 -> Logical_newline_Operator/2

== system Roll_Autopilot_PP/Roll_Autopilot_RollAutopilotSpec1/xxRollAutopilotSpec_31_operator ==
  A : Inport
  B : Inport  Port=2
  Logical_newline_Operator : Logic  Operator=OR  AllPortsSameDT=off  OutDataTypeStr=boolean
  Logical_newline_Operator1 : Logic  Operator=NOT  AllPortsSameDT=off  OutDataTypeStr=boolean
  A_equal__equal__gt_B : Outport  VectorParamsAs1DForOutWhenUnconnected=off
  wires:
  Logical_newline_Operator1/1 -> Logical_newline_Operator/1
  Logical_newline_Operator/1 -> A_equal__equal__gt_B/1
  A/1 -> Logical_newline_Operator1/1
  B/1 -> Logical_newline_Operator/2

== system Roll_Autopilot_PP/Roll_Autopilot_RollAutopilotSpec1/xxRollAutopilotSpec_36_operator ==
  A : Inport
  B : Inport  Port=2
  Logical_newline_Operator : Logic  Operator=OR  AllPortsSameDT=off  OutDataTypeStr=boolean
  Logical_newline_Operator1 : Logic  Operator=NOT  AllPortsSameDT=off  OutDataTypeStr=boolean
  A_equal__equal__gt_B : Outport  VectorParamsAs1DForOutWhenUnconnected=off
  wires:
  Logical_newline_Operator1/1 -> Logical_newline_Operator/1
  Logical_newline_Operator/1 -> A_equal__equal__gt_B/1
  A/1 -> Logical_newline_Operator1/1
  B/1 -> Logical_newline_Operator/2

== system Roll_Autopilot_PP/Roll_Autopilot_RollAutopilotSpec1/xxRollAutopilotSpec_48_operator ==
  A : Inport
  B : Inport  Port=2
  Logical_newline_Operator : Logic  Operator=OR  AllPortsSameDT=off  OutDataTypeStr=boolean
  Logical_newline_Operator1 : Logic  Operator=NOT  AllPortsSameDT=off  OutDataTypeStr=boolean
  A_equal__equal__gt_B : Outport  VectorParamsAs1DForOutWhenUnconnected=off
  wires:
  Logical_newline_Operator1/1 -> Logical_newline_Operator/1
  Logical_newline_Operator/1 -> A_equal__equal__gt_B/1
  A/1 -> Logical_newline_Operator1/1
  B/1 -> Logical_newline_Operator/2

== system Roll_Autopilot_PP/Roll_Autopilot_RollAutopilotSpec1/xxRollAutopilotSpec_57_operator ==
  A : Inport
  B : Inport  Port=2
  Logical_newline_Operator : Logic  Operator=OR  AllPortsSameDT=off  OutDataTypeStr=boolean
  Logical_newline_Operator1 : Logic  Operator=NOT  AllPortsSameDT=off  OutDataTypeStr=boolean
  A_equal__equal__gt_B : Outport  VectorParamsAs1DForOutWhenUnconnected=off
  wires:
  Logical_newline_Operator1/1 -> Logical_newline_Operator/1
  Logical_newline_Operator/1 -> A_equal__equal__gt_B/1
  A/1 -> Logical_newline_Operator1/1
  B/1 -> Logical_newline_Operator/2

== system Roll_Autopilot_PP/Roll_Autopilot_RollAutopilotSpec1/xxRollAutopilotSpec_62_operator ==
  A : Inport
  B : Inport  Port=2
  Logical_newline_Operator : Logic  Operator=OR  AllPortsSameDT=off  OutDataTypeStr=boolean
  Logical_newline_Operator1 : Logic  Operator=NOT  AllPortsSameDT=off  OutDataTypeStr=boolean
  A_equal__equal__gt_B : Outport  VectorParamsAs1DForOutWhenUnconnected=off
  wires:
  Logical_newline_Operator1/1 -> Logical_newline_Operator/1
  Logical_newline_Operator/1 -> A_equal__equal__gt_B/1
  A/1 -> Logical_newline_Operator1/1
  B/1 -> Logical_newline_Operator/2

== system Roll_Autopilot_PP/Roll_Autopilot_RollAutopilotSpec1/xxRollAutopilotSpec_6_operator ==
  A : Inport
  B : Inport  Port=2
  Logical_newline_Operator : Logic  Operator=OR  AllPortsSameDT=off  OutDataTypeStr=boolean
  Logical_newline_Operator1 : Logic  Operator=NOT  AllPortsSameDT=off  OutDataTypeStr=boolean
  A_equal__equal__gt_B : Outport  VectorParamsAs1DForOutWhenUnconnected=off
  wires:
  Logical_newline_Operator1/1 -> Logical_newline_Operator/1
  Logical_newline_Operator/1 -> A_equal__equal__gt_B/1
  A/1 -> Logical_newline_Operator1/1
  B/1 -> Logical_newline_Operator/2

== system Roll_Autopilot_PP/Roll_Autopilot_RollAutopilotSpec1/xxRollAutopilotSpec_77_operator ==
  A : Inport
  B : Inport  Port=2
  Logical_newline_Operator : Logic  Operator=OR  AllPortsSameDT=off  OutDataTypeStr=boolean
  Logical_newline_Operator1 : Logic  Operator=NOT  AllPortsSameDT=off  OutDataTypeStr=boolean
  A_equal__equal__gt_B : Outport  VectorParamsAs1DForOutWhenUnconnected=off
  wires:
  Logical_newline_Operator1/1 -> Logical_newline_Operator/1
  Logical_newline_Operator/1 -> A_equal__equal__gt_B/1
  A/1 -> Logical_newline_Operator1/1
  B/1 -> Logical_newline_Operator/2

== system Roll_Autopilot_PP/Roll_Autopilot_RollAutopilotSpec1/xxRollAutopilotSpec_82_operator ==
  A : Inport
  B : Inport  Port=2
  Logical_newline_Operator : Logic  Operator=OR  AllPortsSameDT=off  OutDataTypeStr=boolean
  Logical_newline_Operator1 : Logic  Operator=NOT  AllPortsSameDT=off  OutDataTypeStr=boolean
  A_equal__equal__gt_B : Outport  VectorParamsAs1DForOutWhenUnconnected=off
  wires:
  Logical_newline_Operator1/1 -> Logical_newline_Operator/1
  Logical_newline_Operator/1 -> A_equal__equal__gt_B/1
  A/1 -> Logical_newline_Operator1/1
  B/1 -> Logical_newline_Operator/2

== system Roll_Autopilot_PP/Roll_Autopilot_RollAutopilotSpec1/xxRollAutopilotSpec_87_operator ==
  A : Inport
  B : Inport  Port=2
  Logical_newline_Operator : Logic  Operator=OR  AllPortsSameDT=off  OutDataTypeStr=boolean
  Logical_newline_Operator1 : Logic  Operator=NOT  AllPortsSameDT=off  OutDataTypeStr=boolean
  A_equal__equal__gt_B : Outport  VectorParamsAs1DForOutWhenUnconnected=off
  wires:
  Logical_newline_Operator1/1 -> Logical_newline_Operator/1
  Logical_newline_Operator/1 -> A_equal__equal__gt_B/1
  A/1 -> Logical_newline_Operator1/1
  B/1 -> Logical_newline_Operator/2

== system Roll_Autopilot_PP/Roll_Autopilot_RollAutopilotSpec1/xxRollAutopilotSpec_99_operator ==
  A : Inport
  B : Inport  Port=2
  Logical_newline_Operator : Logic  Operator=OR  AllPortsSameDT=off  OutDataTypeStr=boolean
  Logical_newline_Operator1 : Logic  Operator=NOT  AllPortsSameDT=off  OutDataTypeStr=boolean
  A_equal__equal__gt_B : Outport  VectorParamsAs1DForOutWhenUnconnected=off
  wires:
  Logical_newline_Operator1/1 -> Logical_newline_Operator/1
  Logical_newline_Operator/1 -> A_equal__equal__gt_B/1
  A/1 -> Logical_newline_Operator1/1
  B/1 -> Logical_newline_Operator/2

== system Roll_Autopilot_PP/Roll_Autopilot/BasicRollMode/CmdLimit ==
  In : Inport
  lower : MinMax  Function=max  Inputs=2  OutDataTypeStr=Inherit: Inherit via back propagation
  lower_limit : Constant  Value=-15  OutDataTypeStr=Inherit: Inherit via back propagation  SampleTime=-1
  upper : MinMax  Inputs=2  OutDataTypeStr=Inherit: Inherit via back propagation
  upper_limit : Constant  Value=15  OutDataTypeStr=Inherit: Inherit via back propagation  SampleTime=-1
  Out : Outport  VectorParamsAs1DForOutWhenUnconnected=off
  wires:
  lower/1 -> Out/1
  In/1 -> upper/2
  lower_limit/1 -> lower/2
  upper/1 -> lower/1
  upper_limit/1 -> upper/1

== system Roll_Autopilot_PP/Roll_Autopilot/BasicRollMode/DispLimit ==
  In : Inport
  lower : MinMax  Function=max  Inputs=2  OutDataTypeStr=Inherit: Inherit via back propagation
  lower_limit : Constant  Value=-30  OutDataTypeStr=Inherit: Inherit via back propagation  SampleTime=-1
  upper : MinMax  Inputs=2  OutDataTypeStr=Inherit: Inherit via back propagation
  upper_limit : Constant  Value=30  OutDataTypeStr=Inherit: Inherit via back propagation  SampleTime=-1
  Out : Outport  VectorParamsAs1DForOutWhenUnconnected=off
  wires:
  lower/1 -> Out/1
  In/1 -> upper/2
  lower_limit/1 -> lower/2
  upper/1 -> lower/1
  upper_limit/1 -> upper/1

== system Roll_Autopilot_PP/Roll_Autopilot/BasicRollMode/Model Info ==
  EmptySubsystem : Subsystem  TreatAsAtomicUnit=on

== system Roll_Autopilot_PP/Roll_Autopilot/BasicRollMode/RateLimit ==
  In : Inport
  lower : MinMax  Function=max  Inputs=2  OutDataTypeStr=Inherit: Inherit via back propagation
  lower_limit : Constant  Value=-6  OutDataTypeStr=Inherit: Inherit via back propagation  SampleTime=-1
  upper : MinMax  Inputs=2  OutDataTypeStr=Inherit: Inherit via back propagation
  upper_limit : Constant  Value=6  OutDataTypeStr=Inherit: Inherit via back propagation  SampleTime=-1
  Out : Outport  VectorParamsAs1DForOutWhenUnconnected=off
  wires:
  lower/1 -> Out/1
  In/1 -> upper/2
  lower_limit/1 -> lower/2
  upper/1 -> lower/1
  upper_limit/1 -> upper/1

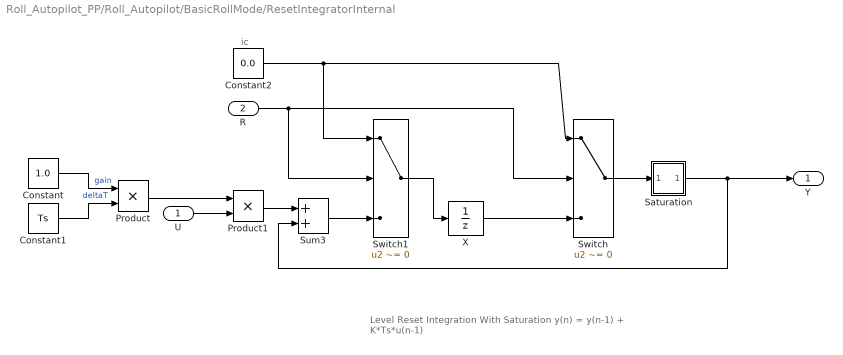
== system Roll_Autopilot_PP/Roll_Autopilot/BasicRollMode/ResetIntegratorInternal ==
  note: ic
  note: Level Reset Integration With Saturation
      | y(n) = y(n-1) + K*Ts*u(n-1)
  U : Inport
  R : Inport  Port=2
  Constant : Constant  Value=1.0
  Constant1 : Constant  Value=Ts
  Constant2 : Constant  Value=0.0
  Product : Product  RndMeth=Zero
  Product1 : Product  RndMeth=Zero
  Saturation : Subsystem  AncestorBlock=pp_lib/saturation  TreatAsAtomicUnit=on
  Sum3 : Sum
  Switch : Switch  Criteria=u2 ~= 0
  Switch1 : Switch  Criteria=u2 ~= 0
  X : UnitDelay  SampleTime=Ts  HasFrameUpgradeWarning=on
  Y : Outport  VectorParamsAs1DForOutWhenUnconnected=off
  wires:
  Product1/1 -> Sum3/1
  U/1 -> Product1/2
  Sum3/1 -> Switch1/3
  Product/1 -> Product1/1
  Switch/1 -> Saturation/1(In)
  Constant2/1 -> Switch1/1, Switch/1
  Constant1/1 -> Product/2  "deltaT"
  Switch1/1 -> X/1
  Constant/1 -> Product/1  "gain"
  Saturation/1(Out) -> Y/1, Sum3/2
  R/1 -> Switch1/2, Switch/2
  X/1 -> Switch/3

== system Roll_Autopilot_PP/Roll_Autopilot/HeadingMode/Model Info ==
  EmptySubsystem : Subsystem  TreatAsAtomicUnit=on

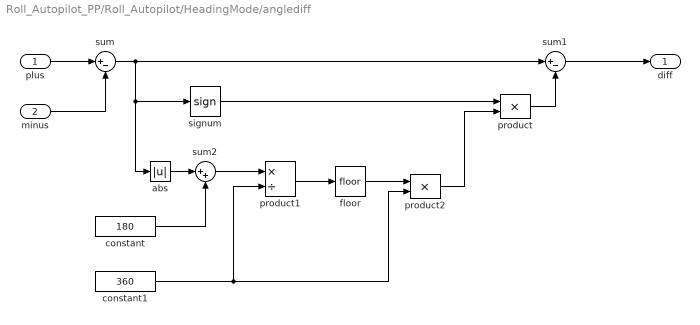
== system Roll_Autopilot_PP/Roll_Autopilot/HeadingMode/anglediff ==
  plus : Inport  OutDataTypeStr=double
  minus : Inport  Port=2  OutDataTypeStr=double
  abs : Abs  ZeroCross=off
  constant : Constant  Value=180
  constant1 : Constant  Value=360
  floor : Rounding
  product : Product  RndMeth=Zero  InputSameDT=on  OutDataTypeStr=Inherit: Same as first input
  product1 : Product  Inputs=*/  RndMeth=Zero  InputSameDT=on  OutDataTypeStr=Inherit: Same as first input
  product2 : Product  RndMeth=Zero  InputSameDT=on  OutDataTypeStr=Inherit: Same as first input
  signum : Signum  ZeroCross=off
  sum : Sum  Inputs=|+-  RndMeth=Zero  InputSameDT=on  OutDataTypeStr=Inherit: Same as first input
  sum1 : Sum  Inputs=|+-  RndMeth=Zero  InputSameDT=on  OutDataTypeStr=Inherit: Same as first input
  sum2 : Sum  Inputs=|++  RndMeth=Zero  InputSameDT=on  OutDataTypeStr=Inherit: Same as first input
  diff : Outport  VectorParamsAs1DForOutWhenUnconnected=off
  wires:
  product2/1 -> product/2
  product/1 -> sum1/2
  sum2/1 -> product1/1
  constant/1 -> sum2/2
  sum1/1 -> diff/1
  signum/1 -> product/1
  floor/1 -> product2/1
  minus/1 -> sum/2
  plus/1 -> sum/1
  product1/1 -> floor/1
  sum/1 -> sum1/1, abs/1, signum/1
  abs/1 -> sum2/1
  constant1/1 -> product2/2, product1/2

== system Roll_Autopilot_PP/Roll_Autopilot/RollReference/latch ==
  note: Xold
  note: Enable
  u : Inport
  E : Inport  Port=2
  Enable : Switch  Criteria=u2 ~= 0  OutDataTypeStr=Inherit: Inherit via back propagation  ZeroCross=off
  FixPt_newline_UnitDelay1 : UnitDelay  SampleTime=Ts
  y : Outport  VectorParamsAs1DForOutWhenUnconnected=off
  wires:
  FixPt_newline_UnitDelay1/1 -> y/1, Enable/3
  Enable/1 -> FixPt_newline_UnitDelay1/1  "Xnew"
  E/1 -> Enable/2
  u/1 -> Enable/1

== system Roll_Autopilot_PP/Roll_Autopilot/BasicRollMode/Model Info/EmptySubsystem ==

== system Roll_Autopilot_PP/Roll_Autopilot/BasicRollMode/ResetIntegratorInternal/Saturation ==
  In : Inport
  lower : MinMax  Function=max  Inputs=2  OutDataTypeStr=Inherit: Inherit via back propagation
  lower_limit : Constant  Value=-5  OutDataTypeStr=Inherit: Inherit via back propagation  SampleTime=-1
  upper : MinMax  Inputs=2  OutDataTypeStr=Inherit: Inherit via back propagation
  upper_limit : Constant  Value=5  OutDataTypeStr=Inherit: Inherit via back propagation  SampleTime=-1
  Out : Outport  VectorParamsAs1DForOutWhenUnconnected=off
  wires:
  lower/1 -> Out/1
  In/1 -> upper/2
  lower_limit/1 -> lower/2
  upper/1 -> lower/1
  upper_limit/1 -> upper/1

== system Roll_Autopilot_PP/Roll_Autopilot/HeadingMode/Model Info/EmptySubsystem ==
